simulink model "lab1"  (R2023b)
settings: Solver=VariableStepAuto  StartTime=0.0  StopTime=30  RelTol=1e-3
model workspace (MAT data in the model file):
  k = 3
  tau = 5
settings Model: Creator=james  LastModifiedBy=jamesvaughan

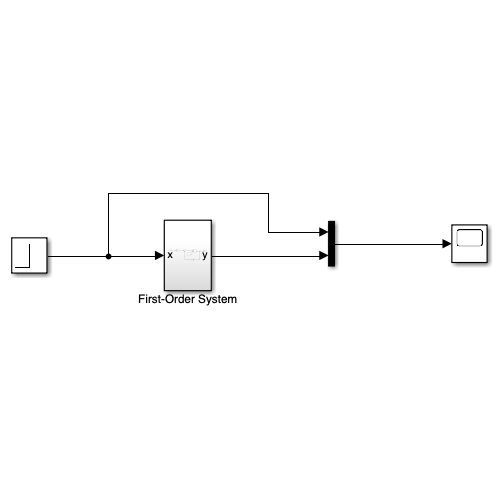
[thumbnail: Simulink's stored preview of the top-level diagram]
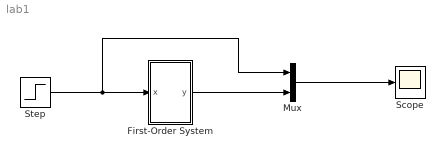
== system lab1 ==
  First-Order System : Subsystem
  Mux : Mux  Inputs=2
  Scope : Scope
  Step : Step  Time=0  SampleTime=0
  wires:
  Step/1 -> Mux/1, First-Order System/1(x)
  Mux/1 -> Scope/1
  First-Order System/1(y) -> Mux/2

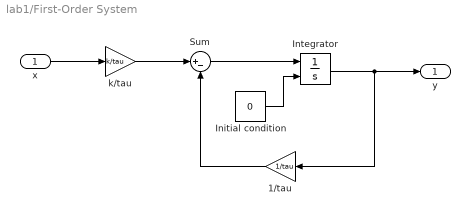
== system lab1/First-Order System ==
  x : Inport
  1/tau : Gain  Gain=1/tau
  Initial condition : Constant  Value=0
  Integrator : Integrator  InitialConditionSource=external
  Sum : Sum  Inputs=|+-
  k/tau : Gain  Gain=k/tau
  y : Outport
  wires:
  Integrator/1 -> 1/tau/1, y/1
  k/tau/1 -> Sum/1
  x/1 -> k/tau/1
  Sum/1 -> Integrator/1
  1/tau/1 -> Sum/2
  Initial condition/1 -> Integrator/2
